simulink model "ESP32_UDP_UART_Bridge"  (R2024b)
settings: Solver=ode4  StartTime=0.0  StopTime=Inf  FixedStep=0.005  RelTol=1e-3  EnableMultiTasking=on
values from neighbouring files (symbols this model uses):
  UDP_DIAG_SOURCE_ID = uint8(1)    [ESP32_UDP_UART_Setup.m]
libraries: arduinowifilib x1, arduinolib x1
(part 1 of 3)
settings Model: ExtModeTrigDuration=2  Creator=mateu  LastModifiedBy=mateu
settings SolverCC: AutoInsertRateTranBlk=on
settings OptimizationCC: EnhancedBackFolding=on  PassReuseOutputArgsAs=Individual arguments  ZeroExternalMemoryAtStartup=off  ZeroInternalMemoryAtStartup=off  MaxStackSize=64  OptimizeBlockOrder=speed  DifferentSizesBufferReuse=on  OptimizationCustomize=off  EfficientTunableParamExpr=on
settings DebuggingCC: ParameterTunabilityLossMsg=error
settings HardwareCC: ProdBitPerPointer=32  ProdBitPerSizeT=32  ProdBitPerPtrDiffT=32  ProdLargestAtomicInteger=Long  ProdLargestAtomicFloat=Double  ProdWordSize=32  ProdHWDeviceType=ARM Compatible->ARM Cortex
settings SFSimCC: MATLABDynamicMemAlloc=off
settings RTWCC: Description=Embedded Coder  SystemTargetFile=ert.tlc  HardwareBoard=ESP32-WROOM(Arduino Compatible)  TLCOptions="-aInlineSetEventsForThisBaseRateFcn=TLC_FALSE -aSuppressMultiTaskScheduler=TLC_FALSE  -aRateBasedStepFcn=0"  TemplateMakefile=ert_default_tmf  Toolchain=ESP32  BuildConfiguration=Faster Runs
settings CodeAppCC: ForceParamTrailComments=on  IgnoreCustomStorageClasses=off  OperatorAnnotations=on  SimulinkDataObjDesc=on  SFDataObjDesc=on  InsertBlockDesc=on
settings ERTTargetCC: SupportContinuousTime=on  SupportVariableSizeSignals=on  ExtModeTransport=3  ExtModeStaticAlloc=on  ExtModeAutomaticAllocSize=off  ExtModeStaticAllocSize=65536  ExtModeMexFile=ext_xcp  ExtModeIntrfLevel=Level2 - Open  InlinedParameterPlacement=Hierarchical

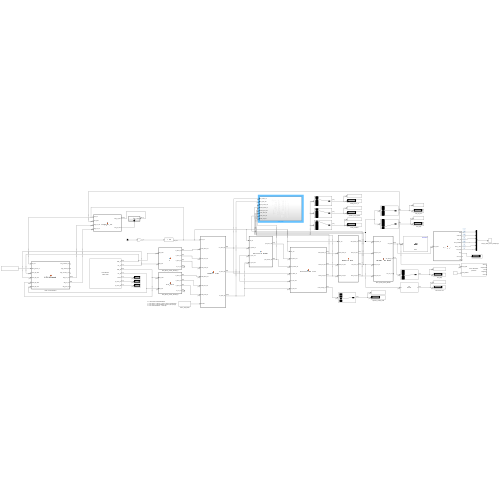
[thumbnail: Simulink's stored preview of the top-level diagram]
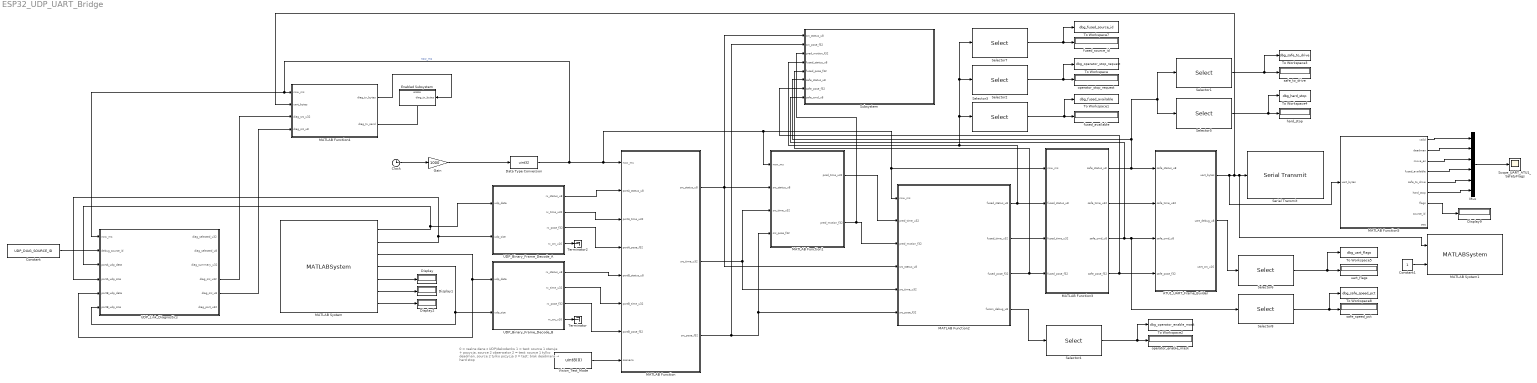
== system ESP32_UDP_UART_Bridge ==
  note: 0 = realne dane z UDP/dekoderów
      | 1 = test: source 1 steruje + pozycja, source 2 obserwator
      | 2 = test: source 1 tylko deadman, source 2 tylko pozycja
      | 3 = test: brak deadmana → hard stop
  ATU1_UART_Frame_Builder : MATLAB Function  TreatAsAtomicUnit=on
  Clock : Clock
  Constant : Constant  Value=UDP_DIAG_SOURCE_ID
  Constant1 : Constant
  Data Type Conversion : DataTypeConversion  OutDataTypeStr=uint32  RndMeth=Floor
  Display{,1..2,9} (4 alike) : Display
  Enabled Subsystem : Subsystem  TreatAsAtomicUnit=on
  Gain : Gain  Gain=1000
  MATLAB Function : MATLAB Function  TreatAsAtomicUnit=on
  MATLAB Function1 : MATLAB Function  TreatAsAtomicUnit=on
  MATLAB Function2 : MATLAB Function  TreatAsAtomicUnit=on
  MATLAB Function3 : MATLAB Function  TreatAsAtomicUnit=on
  MATLAB Function4 : MATLAB Function  TreatAsAtomicUnit=on
  MATLAB Function5 : MATLAB Function  TreatAsAtomicUnit=on
  MATLAB System : MATLABSystem  System=DualUdpReceiverSystem  PortA=uint16( 5005 )  PortB=uint16( 5006 )  MaxPacketSize=uint16( 64 )  SampleTime=0.005  SimulateUsing=Code generation
      mask Type: DualUdpReceiverSystem
      mask Display:
      | disp('Dual UDP RX\n5005 / 5006');
      | port_label('output',1,'data_A');
      | port_label('output',2,'len_A');
      | port_label('output',3,'data_B');
      | port_label('output',4,'len_B');
      | port_label('output',5,'status');
      | port_label('output',6,'rx_count_A');
      | port_label('output',7,'rx_count_B');
  MATLAB System1 : MATLABSystem  System=UartUdpMirrorSystem  PcIp0=uint8(192)  PcIp1=uint8(168)  PcIp2=uint8(0)  PcIp3=uint8(152)  LocalPort=uint16(5010)  RemotePort=uint16(5010)  SampleTime_s=0.02  SimulateUsing=Code generation
      mask Type: UartUdpMirrorSystem
      mask Display:
      | disp('ATU1 UDP Mirror\nport 5010');
      | port_label('input',1,'uart_bytes');
      | port_label('input',2,'send_enable');
      | port_label('output',1,'status');
      | port_label('output',2,'enqueued');
      | port_label('output',3,'sent');
      | port_label('output',4,'dropped');
      | port_label('output',5,'errors');
  Mux : Mux  Inputs=6
  Scope_UART_ATU1_SafetyFlags : Scope
  Selector1 : Selector  InputPortWidth=8  IndexOptions=Index vector (dialog)  Indices=[4]  OutputSizes=1
  Selector2 : Selector  InputPortWidth=8  IndexOptions=Index vector (dialog)  Indices=[2]  OutputSizes=1
  Selector3 : Selector  InputPortWidth=8  IndexOptions=Index vector (dialog)  Indices=[1]  OutputSizes=1
  Selector4 : Selector  InputPortWidth=4  IndexOptions=Index vector (dialog)  Indices=[3]  OutputSizes=1
  Selector5 : Selector  InputPortWidth=8  IndexOptions=Index vector (dialog)  Indices=[7]  OutputSizes=1
  Selector6 : Selector  InputPortWidth=8  IndexOptions=Index vector (dialog)  Indices=[5]  OutputSizes=1
  Selector7 : Selector  InputPortWidth=8  IndexOptions=Index vector (dialog)  Indices=[3]  OutputSizes=1
  Selector8 : Selector  NumberOfDimensions=2  InputPortWidth=4  IndexOptions=Index vector (dialog),Index vector (dialog)  Indices=1,1  OutputSizes=1,1
  Serial Transmit : arduinolib/Serial Transmit  portNumber=2  sendmode=write  sendformat=Decimal  floatprecision=2  header=[]  terminator=[]  blockPlatform=ARDUINO
      settings: SourceProductName=Common
  Subsystem : Subsystem
  Terminator : Terminator
  Terminator2 : Terminator
  To Workspace : ToWorkspace  VariableName=dbg_operator_stop_request  SaveFormat=Timeseries  SampleTime=-1
  To Workspace1 : ToWorkspace  VariableName=dbg_fused_available  SaveFormat=Timeseries  SampleTime=-1
  To Workspace2 : ToWorkspace  VariableName=dbg_operator_enable_mask  SaveFormat=Timeseries  SampleTime=-1
  To Workspace3 : ToWorkspace  VariableName=dbg_safe_to_drive  SaveFormat=Timeseries  SampleTime=-1
  To Workspace4 : ToWorkspace  VariableName=dbg_hard_stop  SaveFormat=Timeseries  SampleTime=-1
  To Workspace5 : ToWorkspace  VariableName=dbg_uart_flags  SaveFormat=Timeseries  SampleTime=-1
  To Workspace7 : ToWorkspace  VariableName=dbg_fused_source_id  SaveFormat=Timeseries  SampleTime=-1
  To Workspace8 : ToWorkspace  VariableName=dbg_safe_speed_pct  SaveFormat=Timeseries  SampleTime=-1
  UDP_Binary_Frame_Decode_A : MATLAB Function  TreatAsAtomicUnit=on
  UDP_Binary_Frame_Decode_B : MATLAB Function  TreatAsAtomicUnit=on
  UDP_Link_Diagnostics : MATLAB Function  TreatAsAtomicUnit=on
  Vision_Test_Mode : Constant  Value=uint8(0)
  fused_available : Display
  fused_source_id : Display
  hard_stop : Display
  operator_enable_mask : Display
  operator_stop_request : Display
  safe_speed_pct : Display
  safe_to_drive : Display
  uart_flags : Display
  wires:
  Clock/1 -> Gain/1
  Gain/1 -> Data Type Conversion/1
  Data Type Conversion/1 -> MATLAB Function4/1(now_ms), UDP_Link_Diagnostics/1(now_ms), MATLAB Function1/1(now_ms), MATLAB Function2/1(now_ms), MATLAB Function3/1(now_ms), MATLAB Function/1(now_ms)  "now_ms"
  UDP_Binary_Frame_Decode_A/1(rx_status_u8) -> MATLAB Function/2(portA_status_u8)
  UDP_Binary_Frame_Decode_A/2(rx_time_u32) -> MATLAB Function/3(portA_time_u32)
  UDP_Binary_Frame_Decode_A/3(rx_pose_f32) -> MATLAB Function/4(portA_pose_f32)
  UDP_Binary_Frame_Decode_B/1(rx_status_u8) -> MATLAB Function/5(portB_status_u8)
  UDP_Binary_Frame_Decode_B/2(rx_time_u32) -> MATLAB Function/6(portB_time_u32)
  UDP_Binary_Frame_Decode_B/3(rx_pose_f32) -> MATLAB Function/7(portB_pose_f32)
  MATLAB Function/1(src_status_u8) -> Subsystem/1(src_status_u8), MATLAB Function1/2(src_status_u8), MATLAB Function2/4(src_status_u8)
  MATLAB Function/2(src_time_u32) -> MATLAB Function1/3(src_time_u32), MATLAB Function2/5(src_time_u32)
  MATLAB Function/3(src_pose_f32) -> Subsystem/2(src_pose_f32), MATLAB Function1/4(src_pose_f32), MATLAB Function2/6(src_pose_f32)
  MATLAB Function1/1(pred_time_u32) -> MATLAB Function2/2(pred_time_u32)
  MATLAB Function1/2(pred_motion_f32) -> Subsystem/3(pred_motion_f32), MATLAB Function2/3(pred_motion_f32)
  MATLAB Function2/3(fused_pose_f32) -> Subsystem/5(fused_pose_f32), MATLAB Function3/4(fused_pose_f32)
  MATLAB Function2/2(fused_time_u32) -> MATLAB Function3/3(fused_time_u32)
  UDP_Binary_Frame_Decode_B/4(rx_crc_u16) -> Terminator/1
  UDP_Binary_Frame_Decode_A/4(rx_crc_u16) -> Terminator2/1
  MATLAB Function3/2(safe_time_u32) -> ATU1_UART_Frame_Builder/2(safe_time_u32)
  MATLAB Function3/1(safe_status_u8) -> ATU1_UART_Frame_Builder/1(safe_status_u8), Subsystem/6(safe_status_u8), Selector1/1, Selector5/1
  Vision_Test_Mode/1 -> MATLAB Function/8(scenario)
  Selector1/1 -> To Workspace3/1, safe_to_drive/1
  Selector2/1 -> To Workspace/1, operator_stop_request/1
  Selector3/1 -> To Workspace1/1, fused_available/1
  Selector4/1 -> To Workspace2/1, operator_enable_mask/1
  MATLAB Function2/4(fusion_debug_u8) -> Selector4/1
  Selector5/1 -> To Workspace4/1, hard_stop/1
  Selector6/1 -> To Workspace5/1, uart_flags/1
  ATU1_UART_Frame_Builder/2(uart_debug_u8) -> Selector6/1
  Selector7/1 -> To Workspace7/1, fused_source_id/1
  MATLAB Function2/1(fused_status_u8) -> MATLAB Function3/2(fused_status_u8), Subsystem/4(fused_status_u8), Selector7/1, Selector2/1, Selector3/1
  Selector8/1 -> To Workspace8/1, safe_speed_pct/1
  Constant/1 -> UDP_Link_Diagnostics/2(debug_source_id)
  MATLAB Function4/1(diag_tx_bytes) -> Enabled Subsystem/1(diag_tx_bytes)
  MATLAB Function4/2(diag_tx_send) -> Enabled Subsystem/Enable
  MATLAB System/1 -> UDP_Binary_Frame_Decode_A/1(udp_data), UDP_Link_Diagnostics/3(portA_udp_data)
  MATLAB System/2 -> UDP_Binary_Frame_Decode_A/2(udp_size), UDP_Link_Diagnostics/4(portA_udp_size)
  MATLAB System/3 -> UDP_Link_Diagnostics/5(portB_udp_data), UDP_Binary_Frame_Decode_B/1(udp_data)
  MATLAB System/4 -> UDP_Link_Diagnostics/6(portB_udp_size), UDP_Binary_Frame_Decode_B/2(udp_size)
  MATLAB System/5 -> Display/1
  MATLAB System/6 -> Display1/1
  MATLAB System/7 -> Display2/1
  UDP_Link_Diagnostics/4(diag_src_u32) -> MATLAB Function4/3(diag_src_u32)
  UDP_Link_Diagnostics/5(diag_src_u8) -> MATLAB Function4/4(diag_src_u8)
  ATU1_UART_Frame_Builder/1(uart_bytes) -> MATLAB System1/1, Serial Transmit/1, MATLAB Function4/2(uart_bytes), MATLAB Function5/1(uart_bytes)
  MATLAB Function5/1(valid) -> Mux/1
  MATLAB Function5/2(deadman) -> Mux/2
  MATLAB Function5/3(move_en) -> Mux/3
  MATLAB Function5/5(safe_to_drive) -> Mux/5
  MATLAB Function5/6(hard_stop) -> Mux/6
  Mux/1 -> Scope_UART_ATU1_SafetyFlags/1
  MATLAB Function5/4(fused_available) -> Mux/4
  MATLAB Function5/7(flags) -> Display9/1
  MATLAB Function3/4(safe_pose_f32) -> ATU1_UART_Frame_Builder/4(safe_pose_f32), Subsystem/7(safe_pose_f32)
  MATLAB Function3/3(safe_cmd_u8) -> Subsystem/8(safe_cmd_u8), ATU1_UART_Frame_Builder/3(safe_cmd_u8), Selector8/1
  Constant1/1 -> MATLAB System1/2

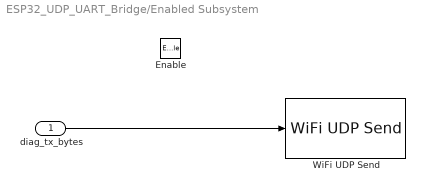
== system ESP32_UDP_UART_Bridge/Enabled Subsystem ==
  diag_tx_bytes : Inport
  Enable : EnablePort
  WiFi UDP Send : arduinowifilib/WiFi UDP Send  remoteIPOctetString=192.168.0.255  remoteport=UDP_DIAG_TARGET_PORT  localport=5007  remoteipoctet1=192  remoteipoctet2=168  remoteipoctet3=0  remoteipoctet4=255  wifiUDPIndex=0  blockPlatform=ARDUINO  isARMArch=false
  wires:
  diag_tx_bytes/1 -> WiFi UDP Send/1

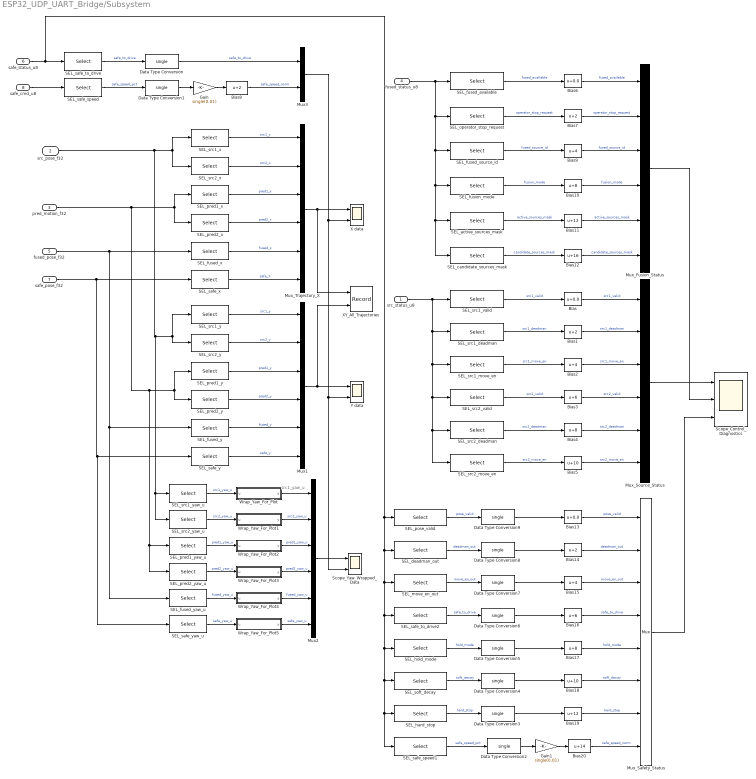
== system ESP32_UDP_UART_Bridge/Subsystem ==
  note: src1_yaw_u
  src_status_u8 : Inport
  src_pose_f32 : Inport  Port=2
  pred_motion_f32 : Inport  Port=3
  fused_status_u8 : Inport  Port=4
  fused_pose_f32 : Inport  Port=5
  safe_status_u8 : Inport  Port=6
  safe_pose_f32 : Inport  Port=7
  safe_cmd_u8 : Inport  Port=8
  Bias : Bias  Bias=0.0  SaturateOnIntegerOverflow=off
  Bias{1,7..8,14} (4 alike) : Bias  Bias=2  SaturateOnIntegerOverflow=off
  Bias10 : Bias  Bias=8  SaturateOnIntegerOverflow=off
  Bias11 : Bias  Bias=12  SaturateOnIntegerOverflow=off
  Bias12 : Bias  Bias=16  SaturateOnIntegerOverflow=off
  Bias13 : Bias  Bias=0.0  SaturateOnIntegerOverflow=off
  Bias15 : Bias  Bias=4  SaturateOnIntegerOverflow=off
  Bias16 : Bias  Bias=6  SaturateOnIntegerOverflow=off
  Bias17 : Bias  Bias=8  SaturateOnIntegerOverflow=off
  Bias18 : Bias  Bias=10  SaturateOnIntegerOverflow=off
  Bias19 : Bias  Bias=12  SaturateOnIntegerOverflow=off
  Bias2 : Bias  Bias=4  SaturateOnIntegerOverflow=off
  Bias20 : Bias  Bias=14  SaturateOnIntegerOverflow=off
  Bias3 : Bias  Bias=6  SaturateOnIntegerOverflow=off
  Bias4 : Bias  Bias=8  SaturateOnIntegerOverflow=off
  Bias5 : Bias  Bias=10  SaturateOnIntegerOverflow=off
  Bias6 : Bias  Bias=0.0  SaturateOnIntegerOverflow=off
  Bias9 : Bias  Bias=4  SaturateOnIntegerOverflow=off
  Data Type Conversion{,1..9} (10 alike) : DataTypeConversion  OutDataTypeStr=single  SaturateOnIntegerOverflow=off  RndMeth=Floor
  Gain : Gain  Gain=single(0.01)
  Gain1 : Gain  Gain=single(0.01)
  Mux1 : Mux  Inputs=6
  Mux2 : Mux  Inputs=6
  Mux3 : Mux  Inputs=2
  Mux_Fusion_Status : Mux  Inputs=6
  Mux_Safety_Status : Mux  Inputs=8
  Mux_Source_Status : Mux  Inputs=6
  Mux_Trajectory_X : Mux  Inputs=6
  SEL_active_sources_mask : Selector  NumberOfDimensions=2  InputPortWidth=3  IndexOptions=Index vector (dialog),Index vector (dialog)  Indices=[7],[1]  OutputSizes=1,1
  SEL_candidate_sources_mask : Selector  NumberOfDimensions=2  InputPortWidth=3  IndexOptions=Index vector (dialog),Index vector (dialog)  Indices=[8],[1]  OutputSizes=1,1
  SEL_deadman_out : Selector  NumberOfDimensions=2  InputPortWidth=3  IndexOptions=Index vector (dialog),Index vector (dialog)  Indices=[2],[1]  OutputSizes=1,1
  SEL_fused_available : Selector  NumberOfDimensions=2  InputPortWidth=3  IndexOptions=Index vector (dialog),Index vector (dialog)  Indices=[1],[1]  OutputSizes=1,1
  SEL_fused_source_id : Selector  NumberOfDimensions=2  InputPortWidth=3  IndexOptions=Index vector (dialog),Index vector (dialog)  Indices=[3],[1]  OutputSizes=1,1
  SEL_fused_x : Selector  NumberOfDimensions=2  InputPortWidth=6  IndexOptions=Index vector (dialog),Index vector (dialog)  Indices=[1],[1]  OutputSizes=1,1
  SEL_fused_y : Selector  NumberOfDimensions=2  InputPortWidth=6  IndexOptions=Index vector (dialog),Index vector (dialog)  Indices=[2],[1]  OutputSizes=1,1
  SEL_fused_yaw_u : Selector  NumberOfDimensions=2  InputPortWidth=6  IndexOptions=Index vector (dialog),Index vector (dialog)  Indices=[5],[1]  OutputSizes=1,1
  SEL_fusion_mode : Selector  NumberOfDimensions=2  InputPortWidth=3  IndexOptions=Index vector (dialog),Index vector (dialog)  Indices=[6],[1]  OutputSizes=1,1
  SEL_hard_stop : Selector  NumberOfDimensions=2  InputPortWidth=3  IndexOptions=Index vector (dialog),Index vector (dialog)  Indices=[7],[1]  OutputSizes=1,1
  SEL_hold_mode : Selector  NumberOfDimensions=2  InputPortWidth=3  IndexOptions=Index vector (dialog),Index vector (dialog)  Indices=[5],[1]  OutputSizes=1,1
  SEL_move_en_out : Selector  NumberOfDimensions=2  InputPortWidth=3  IndexOptions=Index vector (dialog),Index vector (dialog)  Indices=[3],[1]  OutputSizes=1,1
  SEL_operator_stop_request : Selector  NumberOfDimensions=2  InputPortWidth=3  IndexOptions=Index vector (dialog),Index vector (dialog)  Indices=[2],[1]  OutputSizes=1,1
  SEL_pose_valid : Selector  NumberOfDimensions=2  InputPortWidth=3  IndexOptions=Index vector (dialog),Index vector (dialog)  Indices=[1],[1]  OutputSizes=1,1
  SEL_pred1_x : Selector  NumberOfDimensions=2  InputPortWidth=3  IndexOptions=Index vector (dialog),Index vector (dialog)  Indices=[1],[1]  OutputSizes=1,1
  SEL_pred1_y : Selector  NumberOfDimensions=2  InputPortWidth=3  IndexOptions=Index vector (dialog),Index vector (dialog)  Indices=[2],[1]  OutputSizes=1,1
  SEL_pred1_yaw_u : Selector  NumberOfDimensions=2  InputPortWidth=3  IndexOptions=Index vector (dialog),Index vector (dialog)  Indices=[4],[1]  OutputSizes=1,1
  SEL_pred2_x : Selector  NumberOfDimensions=2  InputPortWidth=3  IndexOptions=Index vector (dialog),Index vector (dialog)  Indices=[1],[2]  OutputSizes=1,1
  SEL_pred2_y : Selector  NumberOfDimensions=2  InputPortWidth=3  IndexOptions=Index vector (dialog),Index vector (dialog)  Indices=[2],[2]  OutputSizes=1,1
  SEL_pred2_yaw_u : Selector  NumberOfDimensions=2  InputPortWidth=3  IndexOptions=Index vector (dialog),Index vector (dialog)  Indices=[4],[2]  OutputSizes=1,1
  SEL_safe_speed : Selector  NumberOfDimensions=2  InputPortWidth=3  IndexOptions=Index vector (dialog),Index vector (dialog)  Indices=[1],[1]  OutputSizes=1,1
  SEL_safe_speed1 : Selector  NumberOfDimensions=2  InputPortWidth=3  IndexOptions=Index vector (dialog),Index vector (dialog)  Indices=[1],[1]  OutputSizes=1,1
  SEL_safe_to_drive : Selector  NumberOfDimensions=2  InputPortWidth=3  IndexOptions=Index vector (dialog),Index vector (dialog)  Indices=[4],[1]  OutputSizes=1,1
  SEL_safe_to_drive2 : Selector  NumberOfDimensions=2  InputPortWidth=3  IndexOptions=Index vector (dialog),Index vector (dialog)  Indices=[4],[1]  OutputSizes=1,1
  SEL_safe_x : Selector  NumberOfDimensions=2  InputPortWidth=6  IndexOptions=Index vector (dialog),Index vector (dialog)  Indices=[1],[1]  OutputSizes=1,1
  SEL_safe_y : Selector  NumberOfDimensions=2  InputPortWidth=6  IndexOptions=Index vector (dialog),Index vector (dialog)  Indices=[2],[1]  OutputSizes=1,1
  SEL_safe_yaw_u : Selector  NumberOfDimensions=2  InputPortWidth=6  IndexOptions=Index vector (dialog),Index vector (dialog)  Indices=[5],[1]  OutputSizes=1,1
  SEL_soft_decay : Selector  NumberOfDimensions=2  InputPortWidth=3  IndexOptions=Index vector (dialog),Index vector (dialog)  Indices=[6],[1]  OutputSizes=1,1
  SEL_src1_deadman : Selector  NumberOfDimensions=2  InputPortWidth=3  IndexOptions=Index vector (dialog),Index vector (dialog)  Indices=[4],[1]  OutputSizes=1,1
  SEL_src1_move_en : Selector  NumberOfDimensions=2  InputPortWidth=3  IndexOptions=Index vector (dialog),Index vector (dialog)  Indices=[5],[1]  OutputSizes=1,1
  SEL_src1_valid : Selector  NumberOfDimensions=2  InputPortWidth=3  IndexOptions=Index vector (dialog),Index vector (dialog)  Indices=[3],[1]  OutputSizes=1,1
  SEL_src1_x : Selector  NumberOfDimensions=2  InputPortWidth=3  IndexOptions=Index vector (dialog),Index vector (dialog)  Indices=[1],[1]  OutputSizes=1,1
  SEL_src1_y : Selector  NumberOfDimensions=2  InputPortWidth=3  IndexOptions=Index vector (dialog),Index vector (dialog)  Indices=[2],[1]  OutputSizes=1,1
  SEL_src1_yaw_u : Selector  NumberOfDimensions=2  InputPortWidth=3  IndexOptions=Index vector (dialog),Index vector (dialog)  Indices=[5],[1]  OutputSizes=1,1
  SEL_src2_deadman : Selector  NumberOfDimensions=2  InputPortWidth=3  IndexOptions=Index vector (dialog),Index vector (dialog)  Indices=[4],[2]  OutputSizes=1,1
  SEL_src2_move_en : Selector  NumberOfDimensions=2  InputPortWidth=3  IndexOptions=Index vector (dialog),Index vector (dialog)  Indices=[5],[2]  OutputSizes=1,1
  SEL_src2_valid : Selector  NumberOfDimensions=2  InputPortWidth=3  IndexOptions=Index vector (dialog),Index vector (dialog)  Indices=[3],[2]  OutputSizes=1,1
  SEL_src2_x : Selector  NumberOfDimensions=2  InputPortWidth=3  IndexOptions=Index vector (dialog),Index vector (dialog)  Indices=[1],[2]  OutputSizes=1,1
  SEL_src2_y : Selector  NumberOfDimensions=2  InputPortWidth=3  IndexOptions=Index vector (dialog),Index vector (dialog)  Indices=[2],[2]  OutputSizes=1,1
  SEL_src2_yaw_u : Selector  NumberOfDimensions=2  InputPortWidth=3  IndexOptions=Index vector (dialog),Index vector (dialog)  Indices=[5],[2]  OutputSizes=1,1
  Scope_Control_Diagnostics : Scope  NumInputPorts=3
  Scope_Yaw_Wrapped_Data : Scope  NumInputPorts=2
  Wrap_Yaw_For_Plot : MATLAB Function  TreatAsAtomicUnit=on
  Wrap_Yaw_For_Plot1 : MATLAB Function  TreatAsAtomicUnit=on
  Wrap_Yaw_For_Plot2 : MATLAB Function  TreatAsAtomicUnit=on
  Wrap_Yaw_For_Plot3 : MATLAB Function  TreatAsAtomicUnit=on
  Wrap_Yaw_For_Plot4 : MATLAB Function  TreatAsAtomicUnit=on
  Wrap_Yaw_For_Plot5 : MATLAB Function  TreatAsAtomicUnit=on
  X data : Scope  NumInputPorts=2
  XY_All_Trajectories : Record  FileSettingsInternal="{\"entries\":[{\"content\":{\"excelSettings\":{\"content\":{},\"type\":\"Streamout.ExcelSettings\"}},\"type\":\"Streamout.FileSettingStorage\",\"uuid\":\"\"}],\"packageUris\":[\"http:\\/\\/schema.mathworks.com\\/mf0\\/streamout_blocks\\/R2020a\"],\"version\":\"1.0\"}"  Layout=[1 1]  SignalsInternal="{\"entries\":[{\"content\":{\"signals\":[{\"content\":{\"blockPath\":[],\"dimensions\":[6],\"domain\":\"\",\"hasChildren\":true,\"lineColor\":\"#edb120\",\"lineWidth\":2,\"port\":2,\"sid\":[\"319\"],\"signalID\":1,\"signalName\":\"Mux1\"},\"type\":\"RecordBlkView.Signal\",\"uuid\":\"\"},{\"content\":{\"blockPath\":[],\"channel\":[1],\"dimensions\":[6],\"domain\":\"\",\"lineColor\":\"#64d413\",\"lineWidth\":2,\"parentID\":1,\"plots\":[ 1 ],\"port\":2,\"sid\":[\"319\"],\"signalID\":2,\"signalName\":\"Mux1\"},\"type\":\"RecordBlkView.Signal\",\"uuid\":\"\"},{\"content\":{\"blockPath\":[],\"dimensions\":[6],\"domain\":\"\",\"hasChildren\":true,\"lineColor\":\"#ff6929\",\"lineWidth\":2,\"port\":1,\"sid\":[\"319\"],\"signalID\":3,\"signalName\":\"Mux_Trajectory_X\"},\"type\":\"RecordBlkView.Signal\",\"uuid\":\"\"},{\"content\":{\"blockPath\":[],\"channel\":[1],\"dimensions\":[6],\"domain\":\"\",\"lineColor\":\"#0072bd\",\"lineWidth\":2,\"parentID\":3,\"plots\":[ 1 ],\"port\":1,\"sid\":[\"319\"],\"signalID\":4,\"signalName\":\"Mux_Trajectory_X\"},\"type\":\"RecordBlkView.Signal\",\"uuid\":\"\"},{\"content\":{\"blockPath\":[],\"channel\":[2],\"dimensions\":[6],\"domain\":\"\",\"lineColor\":\"#ff6929\",\"lineWidth\":2,\"parentID\":1,\"plots\":[ 1 ],\"port\":2,\"sid\":[\"319\"],\"signalID\":5,\"signalName\":\"Mux1\"},\"type\":\"RecordBlkView.Signal\",\"uuid\":\"\"},{\"content\":{\"blockPath\":[],\"channel\":[3],\"dimensions\":[6],\"domain\":\"\",\"lineColor\":\"#b746ff\",\"lineWidth\":2,\"parentID\":1,\"plots\":[ 1 ],\"port\":2,\"sid\":[\"319\"],\"signalID\":6,\"signalName\":\"Mux1\"},\"type\":\"RecordBlkView.Signal\",\"uuid\":\"\"},{\"content\":{\"blockPath\":[],\"channel\":[4],\"dimensions\":[6],\"domain\":\"\",\"lineColor\":\"#64d413\",\"lineWidth\":2,\"parentID\":1,\"plots\":[ 1 ],\"port\":2,\"sid\":[\"319\"],\"signalID\":7,\"signalName\":\"Mux1\"},\"type\":\"RecordBlkView.Signal\",\"uuid\":\"\"},{\"content\":{\"blockPath\":[],\"channel\":[5],\"dimensions\":[6],\"domain\":\"\",\"lineColor\":\"#ff13a6\",\"lineWidth\":2,\"parentID\":1,\"plots\":[ 1 ],\"port\":2,\"sid\":[\"319\"],\"signalID\":8,\"signalName\":\"Mux1\"},\"type\":\"RecordBlkView.Signal\",\"uuid\":\"\"},{\"content\":{\"blockPath\":[],\"channel\":[6],\"dimensions\":[6],\"domain\":\"\",\"lineColor\":\"#fe330a\",\"lineWidth\":2,\"parentID\":1,\"plots\":[ 1 ],\"port\":2,\"sid\":[\"319\"],\"signalID\":9,\"signalName\":\"Mux1\"},\"type\":\"RecordBlkView.Signal\",\"uuid\":\"\"},{\"content\":{\"blockPath\":[],\"channel\":[2],\"dimensions\":[6],\"domain\":\"\",\"lineColor\":\"#7e2f8e\",\"lineWidth\":2,\"parentID\":3,\"plots\":[ 1 ],\"port\":1,\"sid\":[\"319\"],\"signalID\":10,\"signalName\":\"Mux_Trajectory_X\"},\"type\":\"RecordBlkView.Signal\",\"uuid\":\"\"},{\"content\":{\"blockPath\":[],\"channel\":[3],\"dimensions\":[6],\"domain\":\"\",\"lineColor\":\"#77ac30\",\"lineWidth\":2,\"parentID\":3,\"plots\":[ 1 ],\"port\":1,\"sid\":[\"319\"],\"signalID\":11,\"signalName\":\"Mux_Trajectory_X\"},\"type\":\"RecordBlkView.Signal\",\"uuid\":\"\"},{\"content\":{\"blockPath\":[],\"channel\":[4],\"dimensions\":[6],\"domain\":\"\",\"lineColor\":\"#4dbeee\",\"lineWidth\":2,\"parentID\":3,\"plots\":[ 1 ],\"port\":1,\"sid\":[\"319\"],\"signalID\":12,\"signalName\":\"Mux_Trajectory_X\"},\"type\":\"RecordBlkView.Signal\",\"uuid\":\"\"},{\"content\":{\"blockPath\":[],\"channel\":[5],\"dimensions\":[6],\"domain\":\"\",\"lineColor\":\"#a2142f\",\"lineWidth\":2,\"parentID\":3,\"plots\":[ 1 ],\"port\":1,\"sid\":[\"319\"],\"signalID\":13,\"signalName\":\"Mux_Trajectory_X\"},\"type\":\"RecordBlkView.Signal\",\"uuid\":\"\"},{\"content\":{\"blockPath\":[],\"channel\":[6],\"dimensions\":[6],\"domain\":\"\",\"lineColor\":\"#139fff\",\"lineWidth\":2,\"parentID\":3,\"plots\":[ 1 ],\"port\":1,\"sid\":[\"319\"],\"signalID\":14,\"signalName\":\"Mux_Trajectory_X\"},\"type\":\"RecordBlkView.Signal\",\"uuid\":\"\"}]},\"type\":\"RecordBlkView.InputSignals\",\"uuid\":\"\"}],\"packageUris\":[\"http:\\/\\/schema.mathworks.com\\/mf0\\/streamout_blocks\\/R2020a\"],\"version\":\"1.0\"}"  VisualizationBindings="{\"xyplotplugin\":{\"info\":[{\"series\":[{\"bindingParametersList\":[{\"parameter\":\"X-Axis\",\"signalID\":4,\"signalName\":\"Mux_Trajectory_X(1)\"},{\"parameter\":\"Y-Axis\",\"signalID\":2,\"signalName\":\"Mux1(1)\"},{\"parameter\":\"X-Axis\",\"signalID\":4,\"signalName\":\"Mux_Trajectory_X(1)\"},{\"parameter\":\"Y-Axis\",\"signalID\":2,\"signalName\":\"Mux1(1)\"}],\"seriesID\":0},{\"bindingParametersList\":[{\"parameter\":\"X-Axis\",\"signalID\":10,\"signalName\":\"Mux_Trajectory_X(2)\"},{\"parameter\":\"Y-Axis\",\"signalID\":5,\"signalName\":\"Mux1(2)\"},{\"parameter\":\"X-Axis\",\"signalID\":10,\"signalName\":\"Mux_Trajectory_X(2)\"},{\"parameter\":\"Y-Axis\",\"signalID\":5,\"signalName\":\"Mux1(2)\"}],\"seriesID\":1},{\"bindingParametersList\":[{\"parameter\":\"X-Axis\",\"signalID\":11,\"signalName\":\"Mux_Trajectory_X(3)\"},{\"parameter\":\"Y-Axis\",\"signalID\":6,\"signalName\":\"Mux1(3)\"},{\"parameter\":\"X-Axis\",\"signalID\":11,\"signalName\":\"Mux_Trajectory_X(3)\"},{\"parameter\":\"Y-Axis\",\"signalID\":6,\"signalName\":\"Mux1(3)\"}],\"seriesID\":2},{\"bindingParametersList\":[{\"parameter\":\"X-Axis\",\"signalID\":12,\"signalName\":\"Mux_Trajectory_X(4)\"},{\"parameter\":\"Y-Axis\",\"signalID\":7,\"signalName\":\"Mux1(4)\"},{\"parameter\":\"X-Axis\",\"signalID\":12,\"signalName\":\"Mux_Trajectory_X(4)\"},{\"parameter\":\"Y-Axis\",\"signalID\":7,\"signalName\":\"Mux1(4)\"}],\"seriesID\":3},{\"bindingParametersList\":[{\"parameter\":\"X-Axis\",\"signalID\":13,\"signalName\":\"Mux_Trajectory_X(5)\"},{\"parameter\":\"Y-Axis\",\"signalID\":8,\"signalName\":\"Mux1(5)\"},{\"parameter\":\"X-Axis\",\"signalID\":13,\"signalName\":\"Mux_Trajectory_X(5)\"},{\"parameter\":\"Y-Axis\",\"signalID\":8,\"signalName\":\"Mux1(5)\"}],\"seriesID\":4},{\"bindingParametersList\":[{\"parameter\":\"X-Axis\",\"signalID\":14,\"signalName\":\"Mux_Trajectory_X(6)\"},{\"parameter\":\"Y-Axis\",\"signalID\":9,\"signalName\":\"Mux1(6)\"},{\"parameter\":\"X-Axis\",\"signalID\":14,\"signalName\":\"Mux_Trajectory_X(6)\"},{\"parameter\":\"Y-Axis\",\"signalID\":9,\"signalName\":\"Mux1(6)\"}],\"seriesID\":5}],\"subplotID\":1}]}}"  CompatibilityTag=XY
  Y data : Scope  NumInputPorts=2
  wires:
  SEL_src1_x/1 -> Mux_Trajectory_X/1  "src1_x"
  SEL_src2_x/1 -> Mux_Trajectory_X/2  "src2_x"
  SEL_pred1_x/1 -> Mux_Trajectory_X/3  "pred1_x"
  SEL_pred2_x/1 -> Mux_Trajectory_X/4  "pred2_x"
  SEL_fused_x/1 -> Mux_Trajectory_X/5  "fused_x"
  Mux_Trajectory_X/1 -> XY_All_Trajectories/1, X data/1
  SEL_src1_y/1 -> Mux1/1  "src1_y"
  Mux1/1 -> XY_All_Trajectories/2, Y data/1
  SEL_pred1_y/1 -> Mux1/3  "pred1_y"
  SEL_pred2_y/1 -> Mux1/4  "pred2_y"
  SEL_fused_y/1 -> Mux1/5  "fused_y"
  SEL_src2_y/1 -> Mux1/2  "src2_y"
  SEL_src1_yaw_u/1 -> Wrap_Yaw_For_Plot/1(u)  "src1_yaw_u"
  src_pose_f32/1 -> SEL_src1_y/1, SEL_src2_y/1, SEL_src1_yaw_u/1, SEL_src2_yaw_u/1, SEL_src2_x/1, SEL_src1_x/1
  fused_pose_f32/1 -> SEL_fused_yaw_u/1, SEL_fused_y/1, SEL_fused_x/1
  Mux2/1 -> Scope_Yaw_Wrapped_Data/1
  SEL_pred1_yaw_u/1 -> Wrap_Yaw_For_Plot2/1(u)  "pred1_yaw_u"
  SEL_pred2_yaw_u/1 -> Wrap_Yaw_For_Plot3/1(u)  "pred2_yaw_u"
  SEL_fused_yaw_u/1 -> Wrap_Yaw_For_Plot4/1(u)  "fused_yaw_u"
  pred_motion_f32/1 -> SEL_pred2_y/1, SEL_pred1_y/1, SEL_pred1_yaw_u/1, SEL_pred2_yaw_u/1, SEL_pred2_x/1, SEL_pred1_x/1
  SEL_src2_yaw_u/1 -> Wrap_Yaw_For_Plot1/1(u)  "src2_yaw_u"
  SEL_safe_x/1 -> Mux_Trajectory_X/6  "safe_X"
  SEL_safe_y/1 -> Mux1/6  "safe_y"
  safe_pose_f32/1 -> SEL_safe_yaw_u/1, SEL_safe_y/1, SEL_safe_x/1
  SEL_safe_yaw_u/1 -> Wrap_Yaw_For_Plot5/1(u)  "safe_yaw_u"
  SEL_safe_to_drive/1 -> Data Type Conversion/1  "safe_to_drive"
  SEL_safe_speed/1 -> Data Type Conversion1/1  "safe_speed_pct"
  safe_cmd_u8/1 -> SEL_safe_speed/1
  Data Type Conversion1/1 -> Gain/1
  Gain/1 -> Bias8/1
  Data Type Conversion/1 -> Mux3/1  "safe_to_drive"
  Mux3/1 -> Y data/2, Scope_Yaw_Wrapped_Data/2, X data/2
  SEL_src1_valid/1 -> Bias/1  "src1_valid"
  SEL_src1_deadman/1 -> Bias1/1  "src1_deadman"
  SEL_src1_move_en/1 -> Bias2/1  "src1_move_en"
  src_status_u8/1 -> SEL_src1_move_en/1, SEL_src2_valid/1, SEL_src2_move_en/1, SEL_src2_deadman/1, SEL_src1_deadman/1, SEL_src1_valid/1
  SEL_src2_deadman/1 -> Bias4/1  "src2_deadman"
  SEL_src2_valid/1 -> Bias3/1  "src2_valid"
  SEL_src2_move_en/1 -> Bias5/1  "src2_move_en"
  Bias4/1 -> Mux_Source_Status/5  "src2_deadman"
  Bias5/1 -> Mux_Source_Status/6  "src2_move_en"
  Bias3/1 -> Mux_Source_Status/4  "src2_valid"
  Bias2/1 -> Mux_Source_Status/3  "src1_move_en"
  Bias1/1 -> Mux_Source_Status/2  "src1_deadman"
  Bias/1 -> Mux_Source_Status/1  "src1_valid"
  Mux_Source_Status/1 -> Scope_Control_Diagnostics/1
  SEL_fused_available/1 -> Bias6/1  "fused_available"
  SEL_operator_stop_request/1 -> Bias7/1  "operator_stop_request"
  Bias8/1 -> Mux3/2  "safe_speed_norm"
  SEL_fusion_mode/1 -> Bias10/1  "fusion_mode"
  SEL_fused_source_id/1 -> Bias9/1  "fused_source_id"
  SEL_candidate_sources_mask/1 -> Bias12/1  "candidate_sources_mask"
  fused_status_u8/1 -> SEL_fused_source_id/1, SEL_candidate_sources_mask/1, SEL_active_sources_mask/1, SEL_fusion_mode/1, SEL_operator_stop_request/1, SEL_fused_available/1
  SEL_active_sources_mask/1 -> Bias11/1  "active_sources_mask"
  Bias6/1 -> Mux_Fusion_Status/1  "fused_available"
  Bias7/1 -> Mux_Fusion_Status/2  "operator_stop_request"
  Bias9/1 -> Mux_Fusion_Status/3  "fused_source_id"
  Bias10/1 -> Mux_Fusion_Status/4  "fusion_mode"
  Bias11/1 -> Mux_Fusion_Status/5  "active_sources_mask"
  Bias12/1 -> Mux_Fusion_Status/6  "candidate_sources_mask"
  Mux_Fusion_Status/1 -> Scope_Control_Diagnostics/2
  SEL_deadman_out/1 -> Data Type Conversion8/1  "deadman_out"
  SEL_hold_mode/1 -> Data Type Conversion5/1  "hold_mode"
  SEL_move_en_out/1 -> Data Type Conversion7/1  "move_en_out"
  SEL_safe_to_drive2/1 -> Data Type Conversion6/1  "safe_to_drive"
  SEL_soft_decay/1 -> Data Type Conversion4/1  "soft_decay"
  SEL_pose_valid/1 -> Data Type Conversion9/1  "pose_valid"
  Bias18/1 -> Mux_Safety_Status/6  "soft_decay"
  Bias15/1 -> Mux_Safety_Status/3  "move_en_out"
  Bias14/1 -> Mux_Safety_Status/2  "deadman_out"
  Bias17/1 -> Mux_Safety_Status/5  "hold_mode"
  Bias16/1 -> Mux_Safety_Status/4  "safe_to_drive"
  Bias13/1 -> Mux_Safety_Status/1  "pose_valid"
  Bias19/1 -> Mux_Safety_Status/7  "hard_stop"
  SEL_hard_stop/1 -> Data Type Conversion3/1  "hard_stop"
  SEL_safe_speed1/1 -> Data Type Conversion2/1  "safe_speed_pct"
  Gain1/1 -> Bias20/1
  Data Type Conversion2/1 -> Gain1/1
  Bias20/1 -> Mux_Safety_Status/8  "safe_speed_norm"
  Data Type Conversion3/1 -> Bias19/1
  Data Type Conversion4/1 -> Bias18/1
  Data Type Conversion5/1 -> Bias17/1
  Data Type Conversion6/1 -> Bias16/1
  Data Type Conversion7/1 -> Bias15/1
  Data Type Conversion8/1 -> Bias14/1
  Data Type Conversion9/1 -> Bias13/1
  safe_status_u8/1 -> SEL_pose_valid/1, SEL_deadman_out/1, SEL_move_en_out/1, SEL_safe_speed1/1, SEL_hard_stop/1, SEL_soft_decay/1, SEL_hold_mode/1, SEL_safe_to_drive2/1, SEL_safe_to_drive/1
  Mux_Safety_Status/1 -> Scope_Control_Diagnostics/3
  Wrap_Yaw_For_Plot/1(y) -> Mux2/1
  Wrap_Yaw_For_Plot1/1(y) -> Mux2/2  "src2_yaw_u"
  Wrap_Yaw_For_Plot2/1(y) -> Mux2/3  "pred1_yaw_u"
  Wrap_Yaw_For_Plot3/1(y) -> Mux2/4  "pred2_yaw_u"
  Wrap_Yaw_For_Plot4/1(y) -> Mux2/5  "fused_yaw_u"
  Wrap_Yaw_For_Plot5/1(y) -> Mux2/6  "safe_yaw_u"

== matlab function ESP32_UDP_UART_Bridge/MATLAB Function1 ==
  data: now_ms input; src_status_u8 input; src_time_u32 input; src_pose_f32 input; pred_time_u32 output; pred_motion_f32 output
% =========================================================
% Vision_Trajectory_Predictor
% =========================================================
% Zadanie:
%   Wyznacza prostą predykcję położenia i orientacji dla każdego
%   źródła Vision source_id=1..4 na podstawie dwóch ostatnich
%   poprawnych pozycji zapisanych w Vision_Source_Memory.
%
% Wejścia:
%   now_ms        : lokalny czas ESP32 w ms, uint32
%   src_status_u8 : status źródeł, 8x4
%   src_time_u32  : czasy źródeł, 5x4
%   src_pose_f32  : ostatnia i poprzednia pozycja źródeł, 10x4
%
% Wyjścia:
%   pred_time_u32, 1x4:
%     1 = pose_age_ms, wiek ostatniej poprawnej pozycji
%
%   pred_motion_f32, 8x4:
%     1 = x_pred
%     2 = y_pred
%     3 = z_pred
%     4 = yaw_unwrapped_pred
%     5 = yaw_deg_pred
%     6 = vx_mps
%     7 = vy_mps
%     8 = vz_mps
%
% Metodyka:
%   Dla każdego źródła, które było widziane i posiada valid pose,
%   blok liczy prędkość liniową z dwóch ostatnich pozycji:
%     vx = (x_last - x_prev) / dt
%     vy = (y_last - y_prev) / dt
%     vz = (z_last - z_prev) / dt
%
%   Następnie przewiduje aktualną pozycję na czas now_ms:
%     x_pred = x_last + vx * age_s
%     y_pred = y_last + vy * age_s
%     z_pred = z_last + vz * age_s
%
%   Yaw przewidywany jest na podstawie yaw_rate_dps z ramki:
%     yaw_unwrapped_pred = yaw_last + yaw_rate_dps * age_s
%
% Uwagi:
%   Jest to predykcja liniowa V1. Nie zawiera jeszcze filtracji
%   prędkości ani ograniczeń dynamiki. Te elementy można dodać później,
%   jeśli logi pokażą zbyt duży szum prędkości.
% =========================================================

function [pred_time_u32, pred_motion_f32] = Vision_Trajectory_Predictor(now_ms, src_status_u8, src_time_u32, src_pose_f32)
%#codegen

pred_time_u32   = zeros(1, 4, 'uint32');
pred_motion_f32 = zeros(8, 4, 'single');

for i = 1:4
    seen     = src_status_u8(1, i);
    has_pose = src_status_u8(2, i);

    if seen ~= 0 && has_pose ~= 0

        last_pose_rx_ms = src_time_u32(4, i);
        prev_pose_rx_ms = src_time_u32(5, i);

        if now_ms >= last_pose_rx_ms
            pose_age_ms = now_ms - last_pose_rx_ms;
        else
            pose_age_ms = uint32(0);
        end

        pred_time_u32(1, i) = pose_age_ms;

        if last_pose_rx_ms > prev_pose_rx_ms
            dt_ms = last_pose_rx_ms - prev_pose_rx_ms;
        else
            dt_ms = uint32(0);
        end

        vx = single(0);
        vy = single(0);
        vz = single(0);

        if dt_ms > 0
            dt_s = single(double(dt_ms) / 1000.0);

            vx = (src_pose_f32(1, i) - src_pose_f32(7, i)) / dt_s;
            vy = (src_pose_f32(2, i) - src_pose_f32(8, i)) / dt_s;
            vz = (src_pose_f32(3, i) - src_pose_f32(9, i)) / dt_s;
        end

        age_s = single(double(pose_age_ms) / 1000.0);

        x_pred = src_pose_f32(1, i) + vx * age_s;
        y_pred = src_pose_f32(2, i) + vy * age_s;
        z_pred = src_pose_f32(3, i) + vz * age_s;

        yaw_unwrapped_pred = src_pose_f32(5, i) + src_pose_f32(6, i) * age_s;
        yaw_deg_pred = wrap_deg_180(yaw_unwrapped_pred);

        pred_motion_f32(1, i) = x_pred;
        pred_motion_f32(2, i) = y_pred;
        pred_motion_f32(3, i) = z_pred;
        pred_motion_f32(4, i) = yaw_unwrapped_pred;
        pred_motion_f32(5, i) = yaw_deg_pred;
        pred_motion_f32(6, i) = vx;
        pred_motion_f32(7, i) = vy;
        pred_motion_f32(8, i) = vz;
    end
end
end

function y = wrap_deg_180(x)
%#codegen

y = x;

while y > single(180.0)
    y = y - single(360.0);
end

while y < single(-180.0)
    y = y + single(360.0);
end
end

== matlab function ESP32_UDP_UART_Bridge/MATLAB Function2 ==
  data: now_ms input; pred_time_u32 input; pred_motion_f32 input; fused_status_u8 output; src_status_u8 input; src_time_u32 input; src_pose_f32 input; fused_time_u32 output; fused_pose_f32 output; fusion_debug_u8 output
function [fused_status_u8, fused_time_u32, fused_pose_f32, fusion_debug_u8] = ...
    Vision_Measurement_Fusion(now_ms, pred_time_u32, pred_motion_f32, src_status_u8, src_time_u32, src_pose_f32)
%#codegen
% =========================================================
% Vision_Measurement_Fusion
% =========================================================
% Zadanie:
%   Wybiera albo łączy pomiary Vision z wielu źródeł source_id=1..4.
%   Blok wykorzystuje dane z Vision_Source_Memory oraz predykcję
%   z Vision_Trajectory_Predictor.
%
% Najważniejsza zasada V2:
%   Autoryzacja jazdy i wybór pomiarów są rozdzielone.
%
%   operator_enable:
%     wystarczy jedno świeże źródło z deadman=1 i move_en=1.
%
%   pose_candidate:
%     źródło musi mieć seen=1, has_pose=1, valid=1, świeżą pozycję
%     i przejść test outlierów. Nie musi mieć własnego deadman=1,
%     jeśli globalnie operator_enable pochodzi z innego telefonu.
%
% Dlaczego tak:
%   Telefon 2 może być tylko obserwatorem albo widzieć tylko tag bazowy.
%   Wtedy może mieć valid=0 i deadman=0, ale nie powinien zatrzymać
%   systemu, jeśli telefon 1 trzyma deadman i ma move_en=1.
%
% Wejścia:
%   now_ms          : lokalny czas ESP32 w ms, uint32
%   pred_time_u32   : 1x4, pose_age_ms dla każdego source_id
%   pred_motion_f32 : 8x4, predykcja pozycji/ruchu
%   src_status_u8   : 8x4, status źródeł
%   src_time_u32    : 5x4, czasy/seq źródeł
%   src_pose_f32    : 10x4, ostatnie dane pozycyjne źródeł
%
% Wyjścia:
%   fused_status_u8, 8x1:
%     1 = fused_available
%     2 = operator_stop_request
%     3 = fused_source_id
%     4 = speed_pct, z najlepszego źródła operator_enable
%     5 = fps_hz, z najlepszego źródła operator_enable
%     6 = fusion_mode, 0=none, 1=single source, 2=weighted fusion
%     7 = active_sources_mask
%     8 = candidate_sources_mask
%
%   fused_time_u32, 3x1:
%     1 = seq najlepszego źródła pozycji
%     2 = unity_t_ms najlepszego źródła pozycji
%     3 = fused_age_ms
%
%   fused_pose_f32, 6x1:
%     1 = x_m
%     2 = y_m
%     3 = z_m
%     4 = yaw_deg
%     5 = yaw_deg_unwrapped
%     6 = yaw_rate_dps
%
%   fusion_debug_u8, 4x1:
%     1 = candidate_count
%     2 = fused_count
%     3 = operator_enable_sources_mask
%     4 = best_control_source_id
% =========================================================

MAX_FRAME_AGE_MS = uint32(250);
MAX_POSE_AGE_MS  = uint32(250);

MAX_FUSE_POS_DIFF_M   = single(0.30);
MAX_FUSE_YAW_DIFF_DEG = single(45.0);

MAX_VEHICLE_SPEED_MPS = single(3.0);
POS_JUMP_MARGIN_M     = single(0.25);
MAX_YAW_JUMP_DEG      = single(120.0);

fused_status_u8 = zeros(8, 1, 'uint8');
fused_time_u32  = zeros(3, 1, 'uint32');
fused_pose_f32  = zeros(6, 1, 'single');
fusion_debug_u8 = zeros(4, 1, 'uint8');

persistent last_fused_valid last_fused_ms
persistent last_x last_y last_z last_yaw_unwrapped

if isempty(last_fused_valid)
    last_fused_valid = uint8(0);
    last_fused_ms = uint32(0);

    last_x = single(0);
    last_y = single(0);
    last_z = single(0);
    last_yaw_unwrapped = single(0);
end

active_sources_mask = uint8(0);
candidate_sources_mask = uint8(0);
operator_enable_sources_mask = uint8(0);

% =========================================================
% 1. Active sources + globalny operator_enable
% =========================================================
% Zasada:
%   Wystarczy jedno świeże źródło z deadman=1 i move_en=1.
%   Nie zatrzymujemy systemu tylko dlatego, że inne źródło ma
%   deadman=0/move_en=0.
%
%   Źródło może dawać operator_enable nawet wtedy, gdy valid=0,
%   np. widzi tylko bazę albo nie ma auta w kadrze.
% =========================================================

best_control_idx = int32(0);
best_control_age = uint32(4294967295);

for i = 1:4
    seen = src_status_u8(1, i);

    if seen ~= 0
        active_sources_mask = bitor(active_sources_mask, bitshift(uint8(1), i - 1));

        last_frame_rx_ms = src_time_u32(3, i);

        if now_ms >= last_frame_rx_ms
            frame_age_ms = now_ms - last_frame_rx_ms;
        else
            frame_age_ms = uint32(0);
        end

        frame_fresh = frame_age_ms <= MAX_FRAME_AGE_MS;

        deadman = src_status_u8(4, i);
        move_en = src_status_u8(5, i);

        if frame_fresh && deadman ~= 0 && move_en ~= 0
            operator_enable_sources_mask = bitor(operator_enable_sources_mask, bitshift(uint8(1), i - 1));

            % Najlepsze źródło sterujące = najświeższy deadman/move_en.
            % Z niego bierzemy speed_pct oraz fps_hz do dalszej ramki.
            if frame_age_ms < best_control_age
                best_control_age = frame_age_ms;
                best_control_idx = int32(i);
            end
        end
    end
end

fused_status_u8(7) = active_sources_mask;
fusion_debug_u8(3) = operator_enable_sources_mask;

if best_control_idx ~= 0
    fusion_debug_u8(4) = uint8(best_control_idx);
end

% Jeśli żadne świeże źródło nie daje deadman=1 i move_en=1,
% to traktujemy to jako globalny stop operatora.
if operator_enable_sources_mask == uint8(0)
    fused_status_u8(2) = uint8(1); % operator_stop_request
    return;
end

% =========================================================
% 2. Kandydaci pozycji
% =========================================================
% Zasada:
%   Kandydat pozycji NIE musi mieć własnego deadman=1.
%   Wystarczy, że globalnie istnieje operator_enable z jakiegoś źródła.
%
%   Kandydat musi mieć:
%     seen=1
%     has_pose=1
%     valid=1
%     pose_age <= MAX_POSE_AGE_MS
%     brak absurdalnego skoku względem ostatniego fused output
% =========================================================

candidate = zeros(1, 4, 'uint8');
candidate_count = uint8(0);

for i = 1:4
    seen     = src_status_u8(1, i);
    has_pose = src_status_u8(2, i);
    valid    = src_status_u8(3, i);

    pose_age_ms = pred_time_u32(1, i);

    logic_ok = seen ~= 0 && has_pose ~= 0 && valid ~= 0;
    fresh_ok = pose_age_ms <= MAX_POSE_AGE_MS;

    outlier_ok = true;

    if last_fused_valid ~= 0
        if now_ms >= last_fused_ms
            dt_since_last_s = single(double(now_ms - last_fused_ms) / 1000.0);
        else
            dt_since_last_s = single(0);
        end

        allowed_pos_jump = POS_JUMP_MARGIN_M + MAX_VEHICLE_SPEED_MPS * dt_since_last_s;

        dx = pred_motion_f32(1, i) - last_x;
        dy = pred_motion_f32(2, i) - last_y;
        dz = pred_motion_f32(3, i) - last_z;

        dist = sqrt(dx*dx + dy*dy + dz*dz);
        yaw_jump = abs(angle_diff_deg(pred_motion_f32(4, i), last_yaw_unwrapped));

        if dist > allowed_pos_jump || yaw_jump > MAX_YAW_JUMP_DEG
            outlier_ok = false;
        end
    end

    if logic_ok && fresh_ok && outlier_ok
        candidate(i) = uint8(1);
        candidate_sources_mask = bitor(candidate_sources_mask, bitshift(uint8(1), i - 1));
        candidate_count = candidate_count + uint8(1);
    end
end

fused_status_u8(8) = candidate_sources_mask;
fusion_debug_u8(1) = candidate_count;

% Jeżeli operator_enable jest, ale nie ma żadnego poprawnego pomiaru,
% to nie robimy stopa tutaj. Zwracamy fused_available=0.
% ESP32_Link_Safety zdecyduje hold/decay/stop na podstawie ostatniego
% dobrego fused state.
if candidate_count == uint8(0)
    return;
end

% =========================================================
% 3. Najlepsze źródło pozycji = najmłodszy kandydat
% =========================================================

best_pose_idx = int32(0);
best_pose_age = uint32(4294967295);

for i = 1:4
    if candidate(i) ~= 0
        if pred_time_u32(1, i) < best_pose_age
            best_pose_age = pred_time_u32(1, i);
            best_pose_idx = int32(i);
        end
    end
end

if best_pose_idx == 0
    return;
end

best = double(best_pose_idx);

best_x = pred_motion_f32(1, best);
best_y = pred_motion_f32(2, best);
best_z = pred_motion_f32(3, best);
best_yaw = pred_motion_f32(4, best);

% =========================================================
% 4. Fuzja ważona źródeł zgodnych z najlepszym
% =========================================================

sum_w = single(0);
sum_x = single(0);
sum_y = single(0);
sum_z = single(0);
sum_yaw = single(0);
sum_yaw_rate = single(0);

fused_count = uint8(0);

for i = 1:4
    if candidate(i) ~= 0

        dx = pred_motion_f32(1, i) - best_x;
        dy = pred_motion_f32(2, i) - best_y;
        dz = pred_motion_f32(3, i) - best_z;

        dist_to_best = sqrt(dx*dx + dy*dy + dz*dz);
        yaw_diff_to_best = abs(angle_diff_deg(pred_motion_f32(4, i), best_yaw));

        if dist_to_best <= MAX_FUSE_POS_DIFF_M && yaw_diff_to_best <= MAX_FUSE_YAW_DIFF_DEG

            age_ratio = single(double(pred_time_u32(1, i)) / double(MAX_POSE_AGE_MS));
            w_age = single(1.0) - age_ratio;

            if w_age < single(0.05)
                w_age = single(0.05);
            end

            w_consistency = single(1.0) - dist_to_best / MAX_FUSE_POS_DIFF_M;

            if w_consistency < single(0.05)
                w_consistency = single(0.05);
            end

            w = w_age * w_consistency;

            yaw_aligned = best_yaw + angle_diff_deg(pred_motion_f32(4, i), best_yaw);

            sum_x = sum_x + w * pred_motion_f32(1, i);
            sum_y = sum_y + w * pred_motion_f32(2, i);
            sum_z = sum_z + w * pred_motion_f32(3, i);
            sum_yaw = sum_yaw + w * yaw_aligned;
            sum_yaw_rate = sum_yaw_rate + w * src_pose_f32(6, i);

            sum_w = sum_w + w;
            fused_count = fused_count + uint8(1);
        end
    end
end

fusion_debug_u8(2) = fused_count;

if sum_w <= single(0)
    return;
end

fused_x = sum_x / sum_w;
fused_y = sum_y / sum_w;
fused_z = sum_z / sum_w;
fused_yaw_unwrapped = sum_yaw / sum_w;
fused_yaw_deg = wrap_deg_180(fused_yaw_unwrapped);
fused_yaw_rate = sum_yaw_rate / sum_w;

% =========================================================
% 5. Wyjścia fused
% =========================================================

control = double(best_control_idx);

fused_status_u8(1) = uint8(1);             % fused_available
fused_status_u8(2) = uint8(0);             % operator_stop_request
fused_status_u8(3) = uint8(best_pose_idx); % fused_source_id = źródło pozycji

% Speed/fps bierzemy z najlepszego źródła operator_enable,
% a niekoniecznie z najlepszego źródła pozycji.
fused_status_u8(4) = src_status_u8(6, control); % speed_pct from control source
fused_status_u8(5) = src_status_u8(7, control); % fps_hz from control source

if fused_count > 1
    fused_status_u8(6) = uint8(2);         % weighted fusion
else
    fused_status_u8(6) = uint8(1);         % single source
end

fused_status_u8(7) = active_sources_mask;
fused_status_u8(8) = candidate_sources_mask;

% Czas/seq bierzemy z najlepszego źródła pozycji.
fused_time_u32(1) = src_time_u32(1, best); % seq
fused_time_u32(2) = src_time_u32(2, best); % unity_t_ms
fused_time_u32(3) = best_pose_age;         % fused_age_ms

fused_pose_f32(1) = fused_x;
fused_pose_f32(2) = fused_y;
fused_pose_f32(3) = fused_z;
fused_pose_f32(4) = fused_yaw_deg;
fused_pose_f32(5) = fused_yaw_unwrapped;
fused_pose_f32(6) = fused_yaw_rate;

last_fused_valid = uint8(1);
last_fused_ms = now_ms;

last_x = fused_x;
last_y = fused_y;
last_z = fused_z;
last_yaw_unwrapped = fused_yaw_unwrapped;
end

function d = angle_diff_deg(a, b)
%#codegen

d = a - b;

while d > single(180.0)
    d = d - single(360.0);
end

while d < single(-180.0)
    d = d + single(360.0);
end
end

function y = wrap_deg_180(x)
%#codegen

y = x;

while y > single(180.0)
    y = y - single(360.0);
end

while y < single(-180.0)
    y = y + single(360.0);
end
end
